simulink model "fir_filter_mac1"  (R2018a)
settings: Solver=VariableStepAuto  StartTime=0.0  StopTime=1e-6  RelTol=1e-3
libraries: xbsIndex_r4 x42
settings Model: Creator=ESPINO NOTEBOOK  LastModifiedBy=ESPINO NOTEBOOK

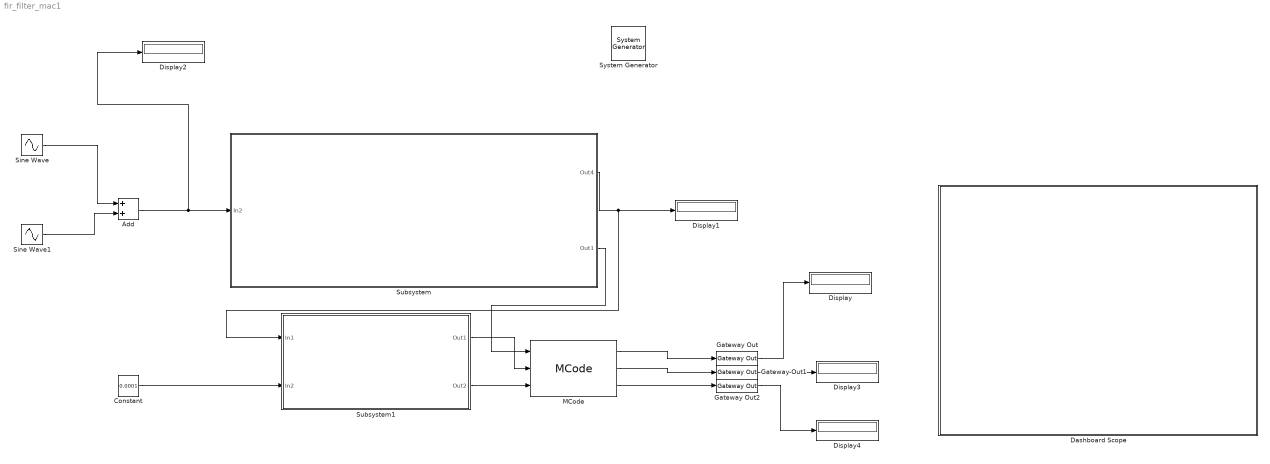
== system fir_filter_mac1 ==
  " System Generator" : xbsIndex_r4/ System Generator  Tag=genX  xilinxfamily=kintex7  part=xc7k325t  speed=-3  package=fbg676  synthesis_tool=Vivado  clock_wrapper=Clock Enables  directory=./netlist  proj_type=Vivado  Synth_file=Vivado Synthesis Defaults  Impl_file=Vivado Implementation Defaults  testbench=on  simulink_period=50e-9  sysclk_period=10  dcm_input_clock_period=10  incr_netlist=off  trim_vbits=Everywhere in SubSystem  dbl_ovrd=According to Block Masks  core_generation=According to Block Masks  run_coregen=off  deprecated_control=off  eval_field=0  block_type=sysgen
  Add : Sum
  Constant : Constant  Value=0.0001
  Dashboard Scope : Subsystem  DialogController=hmiCreateDDGDialog  IsWebBlock=on  mask(MWDashboardBlock){webBlockId=0fb9810e-8db5-4690-99d0-6191defd9f1d, webBlockType=sdiscope, ShowInitialText=on, HMISrcModelName=fir_filter_mac1}
      mask prompts: webBlockId "WebBlock Id"; webBlockType "WebBlock Type"; HMISrcModelName "Source Model"
      mask help: SimulinkHMI:dialogs:HMIScopeDialogDesc
      mask Help: helpview([docroot '/mapfiles/simulink.map'], 'hmi_scope')
      mask Display:
      | if strcmp(get_param(bdroot(gcb),'BlockDiagramType'), 'library')
      |     image([(matlabroot) '/toolbox/simulink/hmi/icons/DashboardScope.png']);
      | end
  Display{,1..4} (5 alike) : Display
  Gateway Out : xbsIndex_r4/Gateway Out  inherit_from_input=off  hdl_port=on  rows=1  columns=1  UseAsDAC=off  DACChannel='1'  interface=None  automatic_assignment=on  address_offset=hex2dec('00')  intf_name=''  intf_description=''  timing_constraint=None  locs_specified=off  LOCs={}  io_standard={}  block_type=gatewayout
  Gateway Out1 : xbsIndex_r4/Gateway Out  inherit_from_input=off  hdl_port=on  rows=1  columns=1  UseAsDAC=off  DACChannel='1'  interface=None  automatic_assignment=on  address_offset=hex2dec('00')  intf_name=''  intf_description=''  timing_constraint=None  locs_specified=off  LOCs={}  io_standard={}  block_type=gatewayout
  Gateway Out2 : xbsIndex_r4/Gateway Out  inherit_from_input=off  hdl_port=on  rows=1  columns=1  UseAsDAC=off  DACChannel='1'  interface=None  automatic_assignment=on  address_offset=hex2dec('00')  intf_name=''  intf_description=''  timing_constraint=None  locs_specified=off  LOCs={}  io_standard={}  block_type=gatewayout
  MCode : xbsIndex_r4/MCode  mfname=xlmax  explicit_period=off  period=1  enable_stdout=off  enable_debug=off  suppress_output=on  defparams={}  hide_port_list={}  dbl_ovrd=off  block_type=mcode
  Sine Wave : Sin  Frequency=2*pi*9e6  SampleTime=0
  Sine Wave1 : Sin  Frequency=2*pi*1e6  SampleTime=0
  Subsystem : Subsystem
  Subsystem1 : Subsystem
  wires:
  Sine Wave/1 -> Add/1
  Sine Wave1/1 -> Add/2
  Add/1 -> Subsystem/1(In2), Display2/1
  Subsystem/1(Out4) -> Subsystem1/1(In1), Display1/1
  Subsystem/2(Out1) -> MCode/1
  MCode/2 -> Gateway Out1/1
  MCode/1 -> Gateway Out/1
  Gateway Out1/1 -> Display3/1
  Gateway Out/1 -> Display/1
  Gateway Out2/1 -> Display4/1
  MCode/3 -> Gateway Out2/1
  Constant/1 -> Subsystem1/2(In2)
  Subsystem1/1(Out1) -> MCode/2
  Subsystem1/2(Out2) -> MCode/3

== system fir_filter_mac1/Dashboard Scope ==

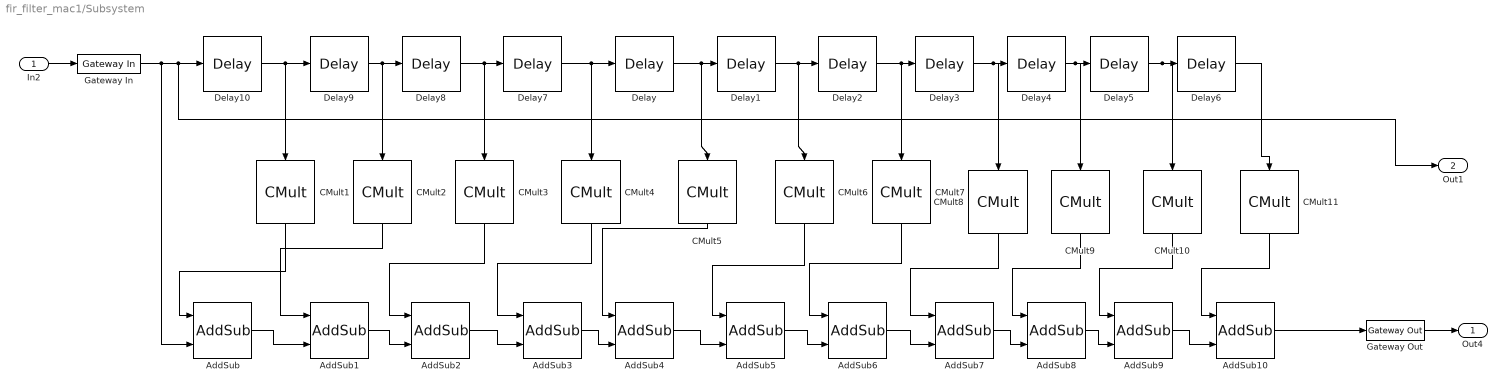
== system fir_filter_mac1/Subsystem ==
  In2 : Inport  SampleTime=50e-9
  AddSub{,1..10} (11 alike) : xbsIndex_r4/AddSub  mode=Addition  use_carryin=off  use_carryout=off  en=off  latency=0  precision=Full  arith_type=Unsigned  n_bits=16  bin_pt=14  quantization=Truncate  overflow=Wrap  use_behavioral_HDL=off  hw_selection=Fabric  pipelined=off  dbl_ovrd=off  block_type=addsub
  CMult1 : xbsIndex_r4/CMult  const=0  gui_display_data_type=Fixed-point  const_n_bits=16  const_bin_pt=14  float_type=Single  exp_bits=8  fraction_bits=24  en=off  latency=0  precision=Full  arith_type="Signed  (2's comp)"  n_bits=16  bin_pt=14  quantization=Truncate  overflow=Wrap  use_behavioral_HDL=off  mem_type=Distributed RAM  pipeline=off  dbl_ovrd=off  block_type=cmult
  CMult10 : xbsIndex_r4/CMult  const=-0.0253  gui_display_data_type=Fixed-point  const_n_bits=16  const_bin_pt=12  float_type=Single  exp_bits=8  fraction_bits=24  en=off  latency=0  precision=Full  arith_type="Signed  (2's comp)"  n_bits=16  bin_pt=14  quantization=Truncate  overflow=Wrap  use_behavioral_HDL=off  mem_type=Distributed RAM  pipeline=off  dbl_ovrd=off  block_type=cmult
  CMult{3,5,7,9,11} (5 alike) : xbsIndex_r4/CMult  const=0  gui_display_data_type=Fixed-point  const_n_bits=16  const_bin_pt=14  float_type=Single  exp_bits=8  fraction_bits=24  en=off  latency=1  precision=Full  arith_type="Signed  (2's comp)"  n_bits=16  bin_pt=14  quantization=Truncate  overflow=Wrap  use_behavioral_HDL=off  mem_type=Distributed RAM  pipeline=off  dbl_ovrd=off  block_type=cmult
  CMult2 : xbsIndex_r4/CMult  const=1  gui_display_data_type=Fixed-point  const_n_bits=18  const_bin_pt=16  float_type=Single  exp_bits=8  fraction_bits=24  en=off  latency=0  precision=Full  arith_type="Signed  (2's comp)"  n_bits=16  bin_pt=14  quantization=Truncate  overflow=Wrap  use_behavioral_HDL=off  mem_type=Distributed RAM  pipeline=off  dbl_ovrd=off  block_type=cmult
  CMult4 : xbsIndex_r4/CMult  const=-0.1271  gui_display_data_type=Fixed-point  const_n_bits=16  const_bin_pt=12  float_type=Single  exp_bits=8  fraction_bits=24  en=off  latency=0  precision=Full  arith_type="Signed  (2's comp)"  n_bits=16  bin_pt=14  quantization=Truncate  overflow=Wrap  use_behavioral_HDL=off  mem_type=Distributed RAM  pipeline=off  dbl_ovrd=off  block_type=cmult
  CMult6 : xbsIndex_r4/CMult  const=0.7965  gui_display_data_type=Fixed-point  const_n_bits=16  const_bin_pt=12  float_type=Single  exp_bits=8  fraction_bits=24  en=off  latency=0  precision=Full  arith_type="Signed  (2's comp)"  n_bits=16  bin_pt=14  quantization=Truncate  overflow=Wrap  use_behavioral_HDL=off  mem_type=Distributed RAM  pipeline=off  dbl_ovrd=off  block_type=cmult
  CMult8 : xbsIndex_r4/CMult  const=-0.1271  gui_display_data_type=Fixed-point  const_n_bits=16  const_bin_pt=12  float_type=Single  exp_bits=8  fraction_bits=24  en=off  latency=0  precision=Full  arith_type="Signed  (2's comp)"  n_bits=16  bin_pt=14  quantization=Truncate  overflow=Wrap  use_behavioral_HDL=off  mem_type=Distributed RAM  pipeline=off  dbl_ovrd=off  block_type=cmult
  Delay{,1..10} (11 alike) : xbsIndex_r4/Delay  rst=off  infoeditControl=Selection of Reset will increase slice count due to use of real FFs and instead of SRLs  en=off  latency=1  reg_retiming=off  dbl_ovrd=off  block_type=delay
  Gateway In : xbsIndex_r4/Gateway In  gui_display_data_type=Fixed-point  arith_type="Signed  (2's comp)"  n_bits=16  bin_pt=12  preci_type=Single  exp_width=8  frac_width=24  rows=1  columns=1  quantization=Truncate  overflow=Wrap  period=50e-9  UseAsADC=off  ADCChannel='1'  interface=None  automatic_assignment=on  address_offset=hex2dec('00')  intf_name=''  intf_description=''  default_value=0  timing_constraint=None  locs_specified=off  LOCs={}  io_standard={}  inherit_from_input=off  hdl_port=on  dbl_ovrd=off  block_type=gatewayin
  Gateway Out : xbsIndex_r4/Gateway Out  inherit_from_input=off  hdl_port=on  rows=1  columns=1  UseAsDAC=off  DACChannel='1'  interface=None  automatic_assignment=on  address_offset=hex2dec('00')  intf_name=''  intf_description=''  timing_constraint=None  locs_specified=off  LOCs={}  io_standard={}  block_type=gatewayout
  Out4 : Outport
  Out1 : Outport  Port=2
  wires:
  CMult1/1 -> AddSub/1
  In2/1 -> Gateway In/1
  Delay/1 -> CMult5/1, Delay1/1
  Delay6/1 -> CMult11/1
  Gateway Out/1 -> Out4/1
  AddSub/1 -> AddSub1/2
  Delay1/1 -> CMult6/1, Delay2/1
  Delay2/1 -> CMult7/1, Delay3/1
  Delay3/1 -> CMult8/1, Delay4/1
  Delay4/1 -> CMult9/1, Delay5/1
  Delay5/1 -> CMult10/1, Delay6/1
  Delay7/1 -> CMult4/1, Delay/1
  Delay8/1 -> CMult3/1, Delay7/1
  Delay9/1 -> CMult2/1, Delay8/1
  Delay10/1 -> CMult1/1, Delay9/1
  CMult2/1 -> AddSub1/1
  AddSub1/1 -> AddSub2/2
  CMult3/1 -> AddSub2/1
  AddSub2/1 -> AddSub3/2
  CMult4/1 -> AddSub3/1
  AddSub3/1 -> AddSub4/2
  CMult5/1 -> AddSub4/1
  CMult6/1 -> AddSub5/1
  AddSub4/1 -> AddSub5/2
  AddSub5/1 -> AddSub6/2
  CMult7/1 -> AddSub6/1
  AddSub6/1 -> AddSub7/2
  CMult8/1 -> AddSub7/1
  AddSub7/1 -> AddSub8/2
  CMult9/1 -> AddSub8/1
  AddSub8/1 -> AddSub9/2
  CMult10/1 -> AddSub9/1
  AddSub9/1 -> AddSub10/2
  CMult11/1 -> AddSub10/1
  Gateway In/1 -> AddSub/2, Out1/1, Delay10/1
  AddSub10/1 -> Gateway Out/1

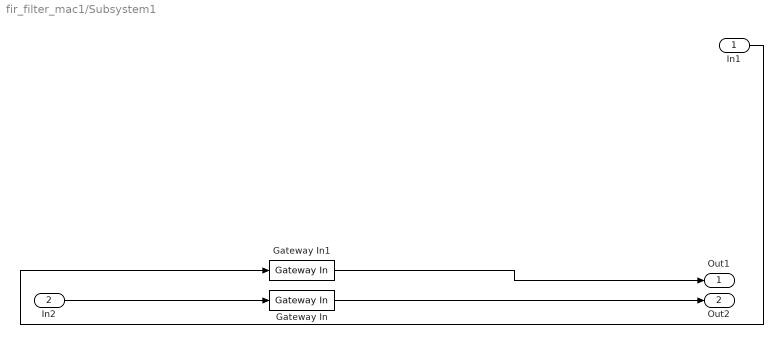
== system fir_filter_mac1/Subsystem1 ==
  In1 : Inport
  In2 : Inport  Port=2
  Gateway In : xbsIndex_r4/Gateway In  gui_display_data_type=Fixed-point  arith_type="Signed  (2's comp)"  n_bits=16  bin_pt=12  preci_type=Single  exp_width=8  frac_width=24  rows=1  columns=1  quantization=Truncate  overflow=Wrap  period=50e-9  UseAsADC=off  ADCChannel='1'  interface=None  automatic_assignment=on  address_offset=hex2dec('00')  intf_name=''  intf_description=''  default_value=0  timing_constraint=None  locs_specified=off  LOCs={}  io_standard={}  inherit_from_input=off  hdl_port=on  dbl_ovrd=off  block_type=gatewayin
  Gateway In1 : xbsIndex_r4/Gateway In  gui_display_data_type=Fixed-point  arith_type="Signed  (2's comp)"  n_bits=16  bin_pt=12  preci_type=Single  exp_width=8  frac_width=24  rows=1  columns=1  quantization=Truncate  overflow=Wrap  period=50e-9  UseAsADC=off  ADCChannel='1'  interface=None  automatic_assignment=on  address_offset=hex2dec('00')  intf_name=''  intf_description=''  default_value=0  timing_constraint=None  locs_specified=off  LOCs={}  io_standard={}  inherit_from_input=off  hdl_port=on  dbl_ovrd=off  block_type=gatewayin
  Out1 : Outport
  Out2 : Outport  Port=2
  wires:
  In1/1 -> Gateway In1/1
  Gateway In1/1 -> Out1/1
  Gateway In/1 -> Out2/1
  In2/1 -> Gateway In/1
